simulink model "mdl"  (R2022a)
settings: Solver=VariableStepAuto  StartTime=0.0  StopTime=10.0  RelTol=1e-3
undefined symbols (not defined in the file): DiscIntNeverNeededParam
settings Model: Creator=whatastarrynight  LastModifiedBy=whatastarrynight

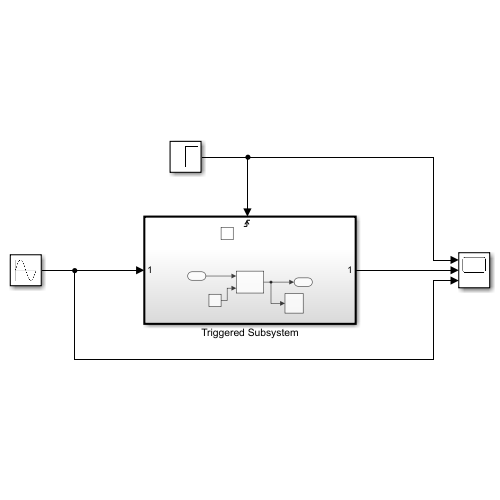
[thumbnail: Simulink's stored preview of the top-level diagram]
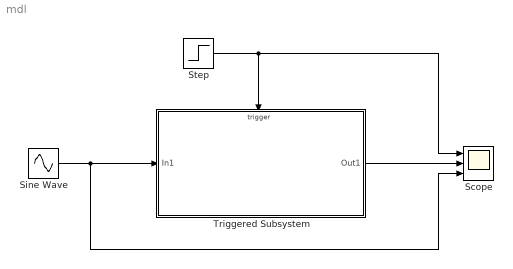
== system mdl ==
  Scope : Scope  NumInputPorts=3
  Sine Wave : Sin  SampleTime=0
  Step : Step  Time=3  SampleTime=0
  Triggered Subsystem : Subsystem  TreatAsAtomicUnit=on
  wires:
  Step/1 -> Scope/1, Triggered Subsystem/Trigger
  Sine Wave/1 -> Scope/3, Triggered Subsystem/1(In1)
  Triggered Subsystem/1(Out1) -> Scope/2

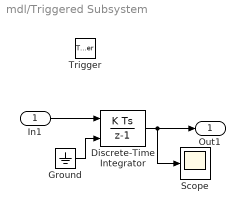
== system mdl/Triggered Subsystem ==
  In1 : Inport
  Trigger : TriggerPort  VariantControl=(inherit)
  Discrete-Time Integrator : DiscreteIntegrator  gainval=1  InitialConditionSource=external  SampleTime=-1  ICPrevOutput=DiscIntNeverNeededParam  ICPrevScaledInput=DiscIntNeverNeededParam
  Ground : Ground
  Scope : Scope
  Out1 : Outport
  wires:
  In1/1 -> Discrete-Time Integrator/1
  Ground/1 -> Discrete-Time Integrator/2
  Discrete-Time Integrator/1 -> Scope/1, Out1/1
